simulink model "Prova_inversione Mixer - NONLINEAR"  (R2015a)
settings: Solver=ode45  StartTime=0.0  StopTime=10.0  RelTol=1e-3
undefined symbols (not defined in the file or in its folder): b, Kq, Kt, m_servo, omega_hover, q_servo, x1
settings Model: Creator=Claudio  LastModifiedBy=Claudio

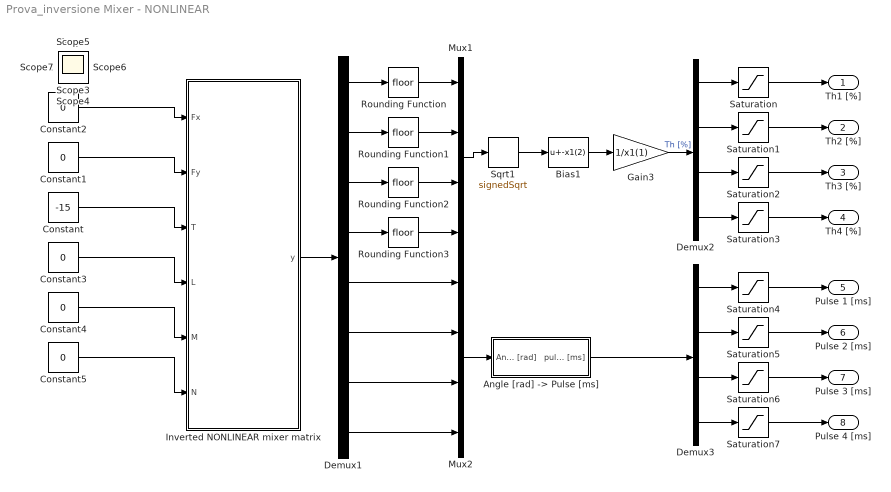
== system Prova_inversione Mixer - NONLINEAR ==
  "Angle [rad] -> Pulse [ms]" : Subsystem
  Bias1 : Bias  Bias=-x1(2)
  Constant : Constant  Value=-15
  Constant{1..5} (5 alike) : Constant  Value=0
  Demux1 : Demux  Outputs=8
  Demux2 : Demux
  Demux3 : Demux
  Gain3 : Gain  Gain=1/x1(1)
  Inverted NONLINEAR mixer matrix : MATLAB Function  TreatAsAtomicUnit=on
  Mux1 : Mux
  Mux2 : Mux
  Rounding Function{,1..3} (4 alike) : Rounding
  Saturation{,1..3} (4 alike) : Saturate  UpperLimit=100  LowerLimit=0
  Saturation{4..7} (4 alike) : Saturate  UpperLimit=2000  LowerLimit=1000
  Sqrt1 : Sqrt  Operator=signedSqrt  SaturateOnIntegerOverflow=on
  Th1 [%] : Outport
  Th2 [%] : Outport  Port=2
  Th3 [%] : Outport  Port=3
  Th4 [%] : Outport  Port=4
  Pulse 1 [ms] : Outport  Port=5
  Pulse 2 [ms] : Outport  Port=6
  Pulse 3 [ms] : Outport  Port=7
  Pulse 4 [ms] : Outport  Port=8
  Scope{,1..7} (8 alike) : Scope
      Scope2 settings: SaveName=ScopeData2
      Scope3 settings: SaveName=ScopeData3
      Scope4 settings: SaveName=ScopeData4
      Scope5 settings: SaveName=ScopeData5
      Scope6 settings: SaveName=ScopeData6
      Scope7 settings: SaveName=ScopeData7
  wires:
  Constant/1 -> Inverted NONLINEAR mixer matrix/3(T)
  Constant1/1 -> Inverted NONLINEAR mixer matrix/2(Fy)
  Constant2/1 -> Inverted NONLINEAR mixer matrix/1(Fx)
  Constant3/1 -> Inverted NONLINEAR mixer matrix/4(L)
  Constant4/1 -> Inverted NONLINEAR mixer matrix/5(M)
  Constant5/1 -> Inverted NONLINEAR mixer matrix/6(N)
  Rounding Function/1 -> Mux1/1
  Saturation6/1 -> Pulse 3 [ms]/1
  Demux3/1 -> Saturation4/1
  Demux3/3 -> Saturation6/1
  Demux1/4 -> Rounding Function3/1
  Demux1/2 -> Rounding Function1/1
  Saturation2/1 -> Th3 [%]/1
  Demux2/2 -> Saturation1/1
  Demux2/1 -> Saturation/1
  Demux2/3 -> Saturation2/1
  Demux2/4 -> Saturation3/1
  Saturation1/1 -> Th2 [%]/1
  Gain3/1 -> Demux2/1  "Th [%]"
  Sqrt1/1 -> Bias1/1
  Mux1/1 -> Sqrt1/1
  Demux1/1 -> Rounding Function/1
  Bias1/1 -> Gain3/1
  Saturation3/1 -> Th4 [%]/1
  Saturation/1 -> Th1 [%]/1
  Demux3/2 -> Saturation5/1
  Rounding Function1/1 -> Mux1/2
  Rounding Function3/1 -> Mux1/4
  Demux1/7 -> Mux2/3
  Demux1/5 -> Mux2/1
  Demux1/6 -> Mux2/2
  Mux2/1 -> "Angle [rad] -> Pulse [ms]"/1(Angle [rad])
  Demux3/4 -> Saturation7/1
  Demux1/3 -> Rounding Function2/1
  Demux1/8 -> Mux2/4
  "Angle [rad] -> Pulse [ms]"/1(pulse [ms]) -> Demux3/1
  Saturation4/1 -> Pulse 1 [ms]/1
  Saturation5/1 -> Pulse 2 [ms]/1
  Saturation7/1 -> Pulse 4 [ms]/1
  Rounding Function2/1 -> Mux1/3
  Inverted NONLINEAR mixer matrix/1(y) -> Demux1/1

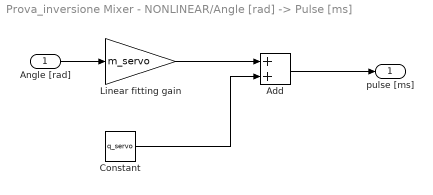
== system Prova_inversione Mixer - NONLINEAR/Angle [rad] -> Pulse [ms] ==
  Angle [rad] : Inport
  Add : Sum
  Constant : Constant  Value=q_servo
  Linear fitting gain : Gain  Gain=m_servo
  pulse [ms] : Outport
  wires:
  Angle [rad]/1 -> Linear fitting gain/1
  Constant/1 -> Add/2
  Linear fitting gain/1 -> Add/1
  Add/1 -> pulse [ms]/1

== matlab function Prova_inversione Mixer - NONLINEAR/Inverted NONLINEAR mixer matrix ==
  data: Fx input; Fy input; T input; L input; M input; N input; y output; omega_hover parameter; Kt parameter; Kq parameter; b parameter
function y = fcn(Fx,Fy,T,L,M,N,omega_hover,Kt,Kq,b)
%#codegen

omega_1 = omega_hover;
omega_2 = omega_hover;
omega_3 = omega_hover;
omega_4 = omega_hover;

% Calcolo prima gli alpha per ottenere la Fx e Fy desiderata considerando
% una omega di hovering
alpha_2 = -asin(Fx/(Kt*(omega_2^2 + omega_4^2)));

alpha_1 = asin(Fy/(Kt*(omega_1^2 + omega_3^2)));
alpha_3 = -alpha_1;
alpha_4 = -alpha_2;

% A questo punto risolvo la matrice K_mix, considerando gli angoli noti e
% risolvo solo per omega_i
K_mix = [
    -Kt*cos(alpha_1),                      -Kt*cos(alpha_2),                    -Kt*cos(alpha_3),                    -Kt*cos(alpha_4);
                                   0, - Kq*sin(alpha_2) - Kt*b*cos(alpha_2),                                   0, Kq*sin(alpha_4) + Kt*b*cos(alpha_4);
 Kt*b*cos(alpha_1) - Kq*sin(alpha_1),                                     0, Kq*sin(alpha_3) - Kt*b*cos(alpha_3),                                   0;
 Kq*cos(alpha_1) + Kt*b*sin(alpha_1),   Kt*b*sin(alpha_2) - Kq*cos(alpha_2), Kq*cos(alpha_3) + Kt*b*sin(alpha_3), Kt*b*sin(alpha_4) - Kq*cos(alpha_4)]

Omega_result = inv(K_mix)*[T;L;M;N];
y = [Omega_result;alpha_1;alpha_2;alpha_3;alpha_4];
